simulink model "exm2_5"  (Simulink 3.00)
settings: Solver=VariableStepDiscrete  SolverMode=SingleTasking  StartTime=0.0  StopTime=10.0  RelTol=1e-3  AbsTol=1e-6
settings Model: RTWTemplateMakefile=grt_vc.tmf

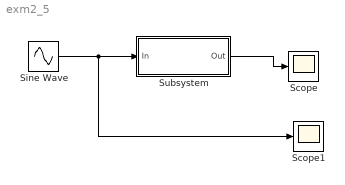
== system exm2_5 ==
  Scope : Scope
      settings: TickLabels=on  TimeRange=auto  YMin=-5  YMax=5  SaveToWorkspace=off  SaveName=ScopeData  DataFormat=Matrix
  Scope1 : Scope
      settings: TickLabels=on  TimeRange=auto  YMin=-5  YMax=5  SaveToWorkspace=off  SaveName=ScopeData  DataFormat=Matrix
  Sine Wave : Sin  Amplitude=1  Frequency=1  Phase=0  SampleTime=0
  Subsystem : Subsystem  mask(comparater){t=0.1}
      mask prompts: t "threshold"
      mask init:
      | th=str2num(t);
      mask StyleString: popup(0.1|0.2|0.3)
      mask Display: disp('The Comparater')
  wires:
  Sine Wave/1 -> Scope1/1, Subsystem/1(In)
  Subsystem/1(Out) -> Scope/1

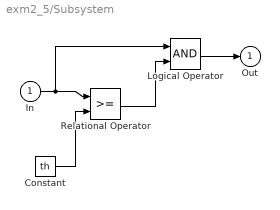
== system exm2_5/Subsystem ==
  In : Inport  Port=1  PortWidth=-1  SampleTime=-1  DataType=auto
      settings: SignalType=auto
  Constant : Constant  Value=th
  Logical Operator : Logic  Operator=AND  Inputs=2
  Relational Operator : RelationalOperator  Operator=>=
  Out : Outport  Port=1  InitialOutput=0
  wires:
  Logical Operator/1 -> Out/1
  In/1 -> Logical Operator/1, Relational Operator/1
  Constant/1 -> Relational Operator/2
  Relational Operator/1 -> Logical Operator/2
